simulink model "Furnace"  (R2020a)
settings: Solver=ode15s  StartTime=0  StopTime=12000  FixedStep=0.1  MaxStep=20  RelTol=1e-08  AbsTol=1e-09
undefined symbols (not defined in the file): k, reg
libraries: simulink x9, mpclib x1
(part 2 of 3)

== system Furnace/Plant/Condenser ==
  F_district : Inport
  F_turb : Inport  Port=2
  T_return : Inport  Port=3
  Constant : Constant  Value=k.cp_water
  Constant1 : Constant  Value=k.epsilon_HE
  Constant2 : Constant  Value=k.eff_HE
  District heating heat exchanger : MATLAB Function  TreatAsAtomicUnit=on
  Scope : Scope
  Transport Delay1 : TransportDelay  DelayTime=2
  Transport Delay2 : TransportDelay  DelayTime=2  InitialOutput=k.T_amb  BufferSize=2048
  Transport Delay3 : TransportDelay  DelayTime=2  InitialOutput=k.T_amb
  Transport Delay4 : TransportDelay  DelayTime=2  InitialOutput=k.T_amb
  p_HP : Constant  Value=k.p_HP
  T_district : Outport  VectorParamsAs1DForOutWhenUnconnected=off
  T_w_out : Outport  Port=2  VectorParamsAs1DForOutWhenUnconnected=off
  F_cond : Outport  Port=3  VectorParamsAs1DForOutWhenUnconnected=off
  wires:
  F_district/1 -> District heating heat exchanger/1(F_DH)
  p_HP/1 -> District heating heat exchanger/2(p_HP)
  T_return/1 -> District heating heat exchanger/4(T_return)
  Constant/1 -> District heating heat exchanger/5(cp_water)
  Constant1/1 -> District heating heat exchanger/6(epsilon_HE)
  District heating heat exchanger/1(Q_HE) -> Transport Delay1/1
  District heating heat exchanger/3(T_district) -> Transport Delay3/1
  District heating heat exchanger/2(Tw_ECO) -> Transport Delay2/1
  F_turb/1 -> Transport Delay4/1, District heating heat exchanger/3(F_turb)
  Transport Delay1/1 -> Scope/1
  Transport Delay2/1 -> T_w_out/1
  Transport Delay3/1 -> T_district/1
  Constant2/1 -> District heating heat exchanger/7(eff_HE)
  Transport Delay4/1 -> F_cond/1

== system Furnace/Plant/Flue-gas fan ==
  T_fg : Inport
  Fi_fg : Inport  Port=2
  Fan : MATLAB Function  TreatAsAtomicUnit=on
  Sum of Elements : Sum  Inputs=+
  Out1 : Outport  VectorParamsAs1DForOutWhenUnconnected=off
  Out2 : Outport  Port=2  VectorParamsAs1DForOutWhenUnconnected=off
  tag scope: W_fan=global
  wires:
  T_fg/1 -> Fan/1(T_fg)
  Sum of Elements/1 -> Fan/2(F_fg)
  Fi_fg/1 -> Out2/1, Sum of Elements/1
  Fan/1(T_out) -> Out1/1
  Fan/2(W_el) -> [W_fan]

== system Furnace/Plant/Flue-gas stack ==
  T_fg : Inport
  Fi_fg : Inport  Port=2
  F_fg : Scope
  T_fg_fromECO : Scope
  wires:
  T_fg/1 -> T_fg_fromECO/1
  Fi_fg/1 -> F_fg/1

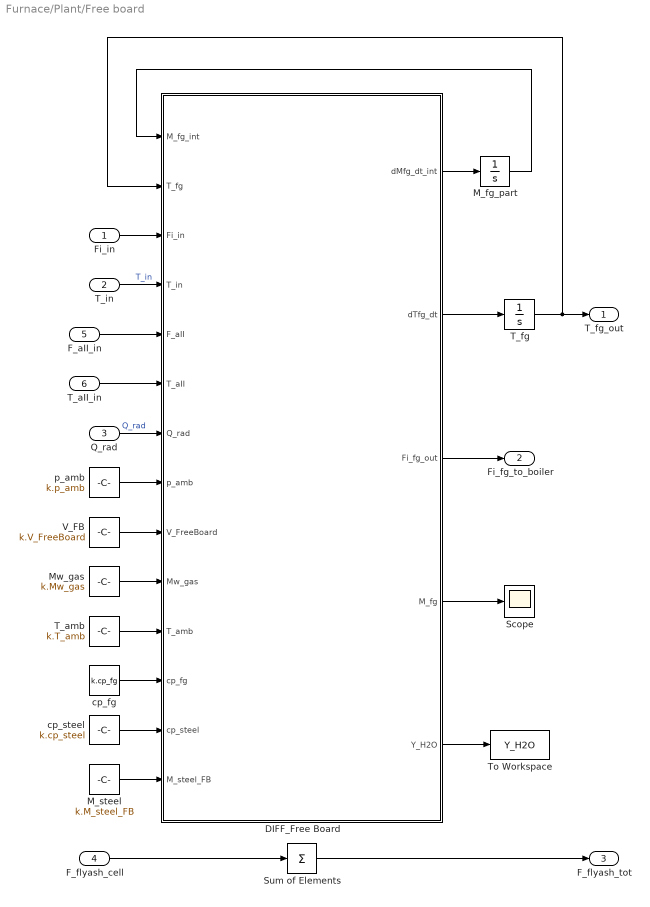
== system Furnace/Plant/Free board ==
  Fi_in : Inport
  T_in : Inport  Port=2
  Q_rad : Inport  Port=3
  F_flyash_cell : Inport  Port=4
  F_aII_in : Inport  Port=5
  T_aII_in : Inport  Port=6
  DIFF_Free Board : MATLAB Function  TreatAsAtomicUnit=on
  M_fg_part : Integrator  InitialCondition=[k.M_fg_IC.*k.w_a(1:k.nc_gas-1)]
  M_steel : Constant  Value=k.M_steel_FB
  Mw_gas : Constant  Value=k.Mw_gas
  Scope : Scope
  Sum of Elements : Sum  Inputs=+
  T_amb : Constant  Value=k.T_amb
  T_fg : Integrator  InitialCondition=k.T_0
  To Workspace : ToWorkspace  VariableName=Y_H2O  SaveFormat=Structure With Time  SampleTime=-1
  V_FB : Constant  Value=k.V_FreeBoard
  cp_fg : Constant  Value=k.cp_fg
  cp_steel : Constant  Value=k.cp_steel
  p_amb : Constant  Value=k.p_amb
  T_fg_out : Outport  VectorParamsAs1DForOutWhenUnconnected=off
  Fi_fg_to_boiler : Outport  Port=2  VectorParamsAs1DForOutWhenUnconnected=off
  F_flyash_tot : Outport  Port=3  VectorParamsAs1DForOutWhenUnconnected=off
  wires:
  T_in/1 -> DIFF_Free Board/4(T_in)  "T_in"
  p_amb/1 -> DIFF_Free Board/8(p_amb)
  DIFF_Free Board/1(dMfg_dt_int) -> M_fg_part/1
  DIFF_Free Board/2(dTfg_dt) -> T_fg/1
  M_fg_part/1 -> DIFF_Free Board/1(M_fg_int)
  DIFF_Free Board/4(M_fg) -> Scope/1
  Q_rad/1 -> DIFF_Free Board/7(Q_rad)  "Q_rad"
  Fi_in/1 -> DIFF_Free Board/3(Fi_in)
  DIFF_Free Board/5(Y_H2O) -> To Workspace/1
  T_fg/1 -> DIFF_Free Board/2(T_fg), T_fg_out/1
  DIFF_Free Board/3(Fi_fg_out) -> Fi_fg_to_boiler/1
  V_FB/1 -> DIFF_Free Board/9(V_FreeBoard)
  Mw_gas/1 -> DIFF_Free Board/10(Mw_gas)
  T_amb/1 -> DIFF_Free Board/11(T_amb)
  cp_fg/1 -> DIFF_Free Board/12(cp_fg)
  cp_steel/1 -> DIFF_Free Board/13(cp_steel)
  M_steel/1 -> DIFF_Free Board/14(M_steel_FB)
  F_flyash_cell/1 -> Sum of Elements/1
  Sum of Elements/1 -> F_flyash_tot/1
  F_aII_in/1 -> DIFF_Free Board/5(F_aII)
  T_aII_in/1 -> DIFF_Free Board/6(T_aII)

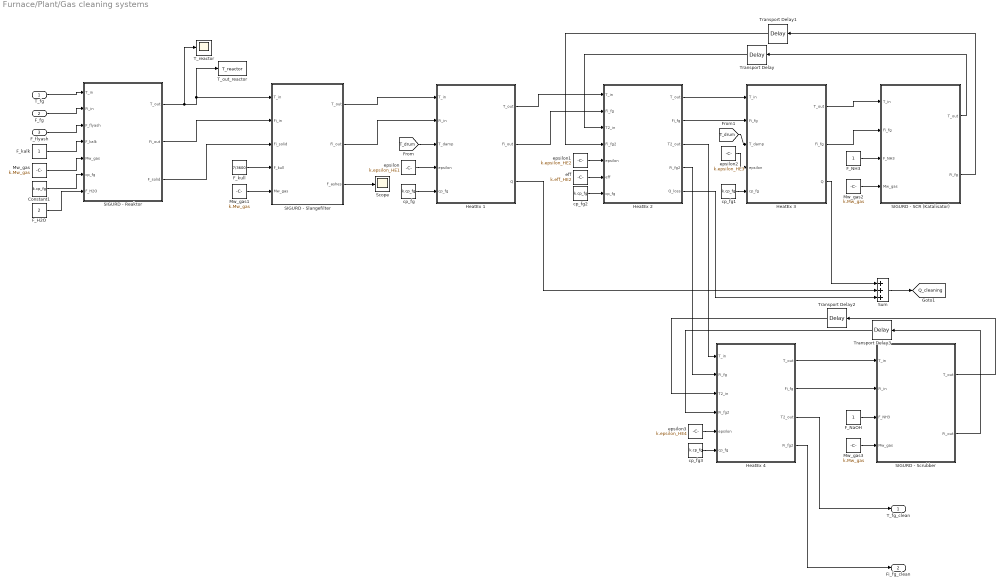
== system Furnace/Plant/Gas cleaning systems ==
  T_fg : Inport
  F_fg : Inport  Port=2
  F_flyash : Inport  Port=3
  Constant1 : Constant  Value=k.cp_fg
  F_H2O : Constant  Value=2
  F_NH3 : Constant
  F_NaOH : Constant
  F_kalk : Constant
  F_kull : Constant  Value=7/3600
  HeatEx 1 : MATLAB Function  TreatAsAtomicUnit=on
  HeatEx 2 : MATLAB Function  TreatAsAtomicUnit=on
  HeatEx 3 : MATLAB Function  TreatAsAtomicUnit=on
  HeatEx 4 : MATLAB Function  TreatAsAtomicUnit=on
  Mw_gas{,1..3} (4 alike) : Constant  Value=k.Mw_gas
  SIGURD - Reaktor : MATLAB Function  TreatAsAtomicUnit=on
  SIGURD - SCR (Katalisator) : MATLAB Function  TreatAsAtomicUnit=on
  SIGURD - Scrubber : MATLAB Function  TreatAsAtomicUnit=on
  SIGURD - Slangefilter : MATLAB Function  TreatAsAtomicUnit=on
  Scope : Scope
  Sum : Sum  Inputs=+++
  T_out_reactor : ToWorkspace  VariableName=T_reactor  SaveFormat=Timeseries  SampleTime=-1
  T_reactor : Scope
  Transport Delay : TransportDelay  DelayTime=2  InitialOutput=k.T_amb
  Transport Delay1 : TransportDelay  DelayTime=2  InitialOutput=ones(k.nc_gas,1)
  Transport Delay2 : TransportDelay  DelayTime=2  InitialOutput=k.T_amb
  Transport Delay3 : TransportDelay  DelayTime=2  InitialOutput=ones(k.nc_gas,1)
  cp_fg{,1..3} (4 alike) : Constant  Value=k.cp_fg
  eff : Constant  Value=k.eff_HE2
  epsilon : Constant  Value=k.epsilon_HE1
  epsilon1 : Constant  Value=k.epsilon_HE2
  epsilon2 : Constant  Value=k.epsilon_HE3
  epsilon3 : Constant  Value=k.epsilon_HE4
  T_fg_clean : Outport  VectorParamsAs1DForOutWhenUnconnected=off
  Fi_fg_clean : Outport  Port=2  VectorParamsAs1DForOutWhenUnconnected=off
  tag scope: Q_cleaning=global
  wires:
  T_fg/1 -> SIGURD - Reaktor/1(T_in)
  F_fg/1 -> SIGURD - Reaktor/2(Fi_in)
  SIGURD - Reaktor/1(T_out) -> T_reactor/1, T_out_reactor/1, SIGURD - Slangefilter/1(T_in)
  SIGURD - Reaktor/2(Fi_out) -> SIGURD - Slangefilter/2(Fi_in)
  F_kalk/1 -> SIGURD - Reaktor/4(F_kalk)
  Mw_gas/1 -> SIGURD - Reaktor/5(Mw_gas)
  F_kull/1 -> SIGURD - Slangefilter/4(F_kull)
  Mw_gas1/1 -> SIGURD - Slangefilter/5(Mw_gas)
  SIGURD - Slangefilter/1(T_out) -> HeatEx 1/1(T_in)
  SIGURD - Slangefilter/2(Fi_out) -> HeatEx 1/2(Fi_in)
  [T_drum] -> HeatEx 1/3(T_damp)
  epsilon/1 -> HeatEx 1/4(epsilon)
  HeatEx 1/1(T_out) -> HeatEx 2/1(T_in)
  HeatEx 1/2(Fi_out) -> HeatEx 2/2("Fi_fg ")
  HeatEx 2/1(T_out) -> HeatEx 3/1(T_in)
  HeatEx 2/2(Fi_fg) -> HeatEx 3/2("Fi_fg ")
  [T_drum] -> HeatEx 3/3(T_damp)
  epsilon1/1 -> HeatEx 2/5(epsilon)
  epsilon2/1 -> HeatEx 3/4(epsilon)
  HeatEx 1/3(Q) -> Sum/2
  HeatEx 3/3(Q) -> Sum/1
  HeatEx 3/1(T_out) -> SIGURD - SCR (Katalisator)/1(T_in)
  HeatEx 3/2(Fi_fg) -> SIGURD - SCR (Katalisator)/2("Fi_fg ")
  F_NH3/1 -> SIGURD - SCR (Katalisator)/3(F_NH3)
  Mw_gas2/1 -> SIGURD - SCR (Katalisator)/4(Mw_gas)
  SIGURD - SCR (Katalisator)/1(T_out) -> Transport Delay/1
  SIGURD - SCR (Katalisator)/2(Fi_fg) -> Transport Delay1/1
  HeatEx 2/3(T2_out) -> HeatEx 4/1(T_in)
  HeatEx 2/4(Fi_fg2) -> HeatEx 4/2("Fi_fg ")
  epsilon3/1 -> HeatEx 4/5(epsilon)
  HeatEx 4/1(T_out) -> SIGURD - Scrubber/1(T_in)
  HeatEx 4/2(Fi_fg) -> SIGURD - Scrubber/2(Fi_in)
  SIGURD - Scrubber/1(T_out) -> Transport Delay2/1
  SIGURD - Scrubber/2(Fi_out) -> Transport Delay3/1
  F_NaOH/1 -> SIGURD - Scrubber/3(F_NH3)
  Mw_gas3/1 -> SIGURD - Scrubber/4(Mw_gas)
  HeatEx 4/3(T2_out) -> T_fg_clean/1
  HeatEx 4/4(Fi_fg2) -> Fi_fg_clean/1
  SIGURD - Slangefilter/3(F_ashes) -> Scope/1
  cp_fg/1 -> HeatEx 1/5(cp_fg)
  cp_fg1/1 -> HeatEx 3/5(cp_fg)
  cp_fg2/1 -> HeatEx 2/7(cp_fg)
  Constant1/1 -> SIGURD - Reaktor/6(cp_fg)
  SIGURD - Reaktor/3(F_solid) -> SIGURD - Slangefilter/3(Fi_solid)
  F_flyash/1 -> SIGURD - Reaktor/3(F_flyash)
  Transport Delay/1 -> HeatEx 2/3(T2_in)
  Transport Delay1/1 -> HeatEx 2/4("Fi_fg2 ")
  Transport Delay2/1 -> HeatEx 4/3(T2_in)
  Transport Delay3/1 -> HeatEx 4/4("Fi_fg2 ")
  cp_fg3/1 -> HeatEx 4/6(cp_fg)
  eff/1 -> HeatEx 2/6(eff)
  Sum/1 -> [Q_cleaning]
  HeatEx 2/5(Q_loss) -> Sum/3
  F_H2O/1 -> SIGURD - Reaktor/7(F_H2O)

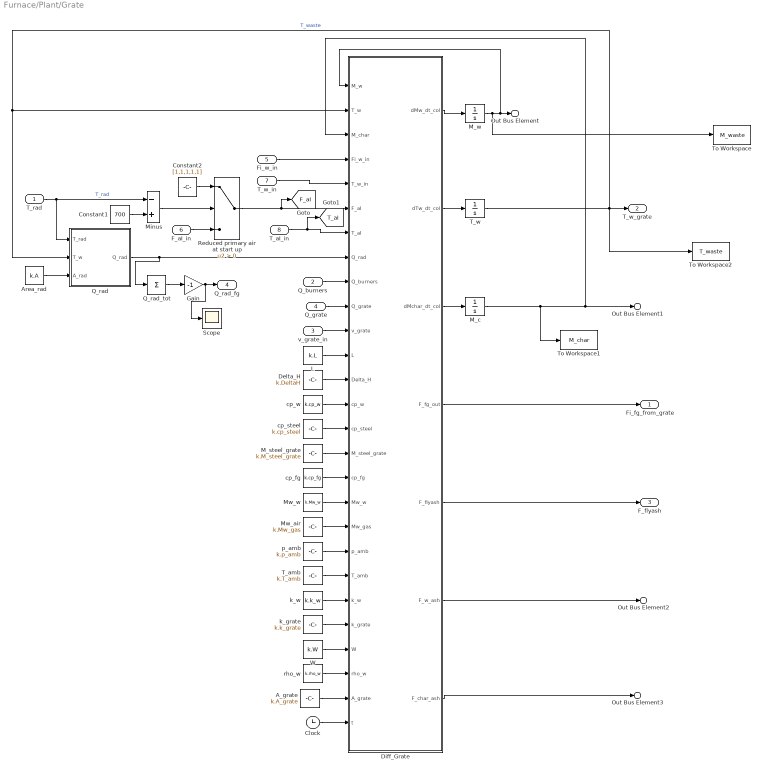
== system Furnace/Plant/Grate ==
  T_rad : Inport
  Q_burners : Inport  Port=2
  v_grate_in : Inport  Port=3
  Q_grate : Inport  Port=4
  Fi_w_in : Inport  Port=5
  F_aI_in : Inport  Port=6
  T_w_in : Inport  Port=7
  T_aI_in : Inport  Port=8
  A_grate : Constant  Value=k.A_grate
  Area_rad : Constant  Value=k.A
  Clock : Clock
  Constant1 : Constant  Value=700
  Constant2 : Constant  Value=[1,1,1,1,1]
  Delta_H : Constant  Value=k.DeltaH
  Diff_Grate : MATLAB Function  TreatAsAtomicUnit=on
  Gain : Gain  Gain=-1
  L : Constant  Value=k.L
  M_c : Integrator  InitialCondition=zeros(k.n_cell,1)
  M_steel_grate : Constant  Value=k.M_steel_grate
  M_w : Integrator  InitialCondition=zeros(k.n_cell.*(k.nc_w+2),1)
  Minus : Sum  Inputs=-+
  Mw_air : Constant  Value=k.Mw_gas
  Mw_w : Constant  Value=k.Mw_w
  Q_rad : Subsystem
  Q_rad_tot : Sum  Inputs=+
  Reduced primary air at start up : Switch  Criteria=u2 > Threshold
  Scope : Scope
  T_amb : Constant  Value=k.T_amb
  T_w : Integrator  InitialCondition=k.T_amb.*ones(k.n_cell,1)
  To Workspace : ToWorkspace  VariableName=M_waste  SaveFormat=Structure With Time  SampleTime=-1
  To Workspace1 : ToWorkspace  VariableName=M_char  SaveFormat=Structure With Time  SampleTime=-1
  To Workspace2 : ToWorkspace  VariableName=T_waste  SaveFormat=Structure With Time  SampleTime=-1
  W : Constant  Value=k.W
  cp_fg : Constant  Value=k.cp_fg
  cp_steel : Constant  Value=k.cp_steel
  cp_w : Constant  Value=k.cp_w
  k_grate : Constant  Value=k.k_grate
  k_w : Constant  Value=k.k_w
  p_amb : Constant  Value=k.p_amb
  rho_w : Constant  Value=k.rho_w
  Fi_fg_from_grate : Outport  VectorParamsAs1DForOutWhenUnconnected=off
  T_w_grate : Outport  Port=2  VectorParamsAs1DForOutWhenUnconnected=off
  F_flyash : Outport  Port=3  VectorParamsAs1DForOutWhenUnconnected=off
  Q_rad_fg : Outport  Port=4  VectorParamsAs1DForOutWhenUnconnected=off
  Out Bus Element : Outport  Port=5  VectorParamsAs1DForOutWhenUnconnected=off  PortName=OutBus  Element=M_w_grate
  Out Bus Element1 : Outport  Port=5  VectorParamsAs1DForOutWhenUnconnected=off  PortName=OutBus  Element=M_char
  Out Bus Element2 : Outport  Port=5  VectorParamsAs1DForOutWhenUnconnected=off  PortName=OutBus  Element=F_w_ash
  Out Bus Element3 : Outport  Port=5  VectorParamsAs1DForOutWhenUnconnected=off  PortName=OutBus  Element=F_char_ash
  tag scope: F_aI=global, T_aI=global
  wires:
  Diff_Grate/2(dTw_dt_col) -> T_w/1
  Area_rad/1 -> Q_rad/3(A_rad)
  M_w/1 -> To Workspace/1, Out Bus Element/1, Diff_Grate/1(M_w)
  T_aI_in/1 -> [T_aI], Diff_Grate/7(T_aI)
  Q_rad/1(Q_rad) -> Q_rad_tot/1, Diff_Grate/8(Q_rad)
  Diff_Grate/1(dMw_dt_col) -> M_w/1
  T_w/1 -> Diff_Grate/2(T_w), Q_rad/2(T_w), T_w_grate/1, To Workspace2/1  "T_waste"
  Diff_Grate/6(F_w_ash) -> Out Bus Element2/1
  Diff_Grate/4(F_fg_out) -> Fi_fg_from_grate/1
  Diff_Grate/3(dMchar_dt_col) -> M_c/1
  M_c/1 -> To Workspace1/1, Out Bus Element1/1, Diff_Grate/3(M_char)
  Diff_Grate/7(F_char_ash) -> Out Bus Element3/1
  Q_rad_tot/1 -> Gain/1
  Gain/1 -> Scope/1, Q_rad_fg/1
  Q_burners/1 -> Diff_Grate/9(Q_burners)
  Clock/1 -> Diff_Grate/27(t)
  Q_grate/1 -> Diff_Grate/10(Q_grate)
  T_rad/1 -> Minus/1, Q_rad/1(T_rad)  "T_rad"
  Constant1/1 -> Minus/2
  Minus/1 -> Reduced primary air at start up/2
  F_aI_in/1 -> Reduced primary air at start up/3
  Reduced primary air at start up/1 -> [F_aI], Diff_Grate/6(F_aI)
  Constant2/1 -> Reduced primary air at start up/1
  L/1 -> Diff_Grate/12(L)
  Delta_H/1 -> Diff_Grate/13(Delta_H)
  cp_w/1 -> Diff_Grate/14(cp_w)
  cp_steel/1 -> Diff_Grate/15(cp_steel)
  M_steel_grate/1 -> Diff_Grate/16(M_steel_grate)
  cp_fg/1 -> Diff_Grate/17(cp_fg)
  Mw_w/1 -> Diff_Grate/18(Mw_w)
  Mw_air/1 -> Diff_Grate/19(Mw_gas)
  p_amb/1 -> Diff_Grate/20(p_amb)
  T_amb/1 -> Diff_Grate/21(T_amb)
  k_w/1 -> Diff_Grate/22(k_w)
  k_grate/1 -> Diff_Grate/23(k_grate)
  W/1 -> Diff_Grate/24(W)
  rho_w/1 -> Diff_Grate/25(rho_w)
  A_grate/1 -> Diff_Grate/26(A_grate)
  Diff_Grate/5(F_flyash) -> F_flyash/1
  v_grate_in/1 -> Diff_Grate/11(v_grate)
  Fi_w_in/1 -> Diff_Grate/4(Fi_w_in)
  T_w_in/1 -> Diff_Grate/5(T_w_in)

== system Furnace/Plant/Hot water to district heating ==
  In1 : Inport
  T_district : Scope
  wires:
  In1/1 -> T_district/1

== system Furnace/Plant/Turbine ==
  T_SH : Inport
  F_SH : Inport  Port=2
  p_drum : Inport  Port=3
  Scope : Scope
  Sum : Sum
  Transport Delay1 : TransportDelay  DelayTime=3
  Transport Delay2 : TransportDelay  DelayTime=3
  Turbine : MATLAB Function  TreatAsAtomicUnit=on
  W_net : Scope
  eta_TURB : Constant  Value=k.eta_TURB
  p_HP : Constant  Value=k.p_HP
  p_LP : Constant  Value=k.p_LP
  F_turb : Outport  VectorParamsAs1DForOutWhenUnconnected=off
  wires:
  T_SH/1 -> Turbine/1(T_SH)
  Turbine/1(W_el) -> Transport Delay1/1
  p_drum/1 -> Turbine/3(p_drum)
  F_SH/1 -> Transport Delay2/1, Turbine/2(F_SH)
  p_LP/1 -> Turbine/5(p_LP)
  Transport Delay1/1 -> Sum/1
  Transport Delay2/1 -> F_turb/1
  p_HP/1 -> Turbine/4(p_HP)
  Turbine/2(Q_turb) -> Scope/1
  eta_TURB/1 -> Turbine/6(eta_TURB)
  [W_fan] -> Sum/2
  Sum/1 -> W_net/1

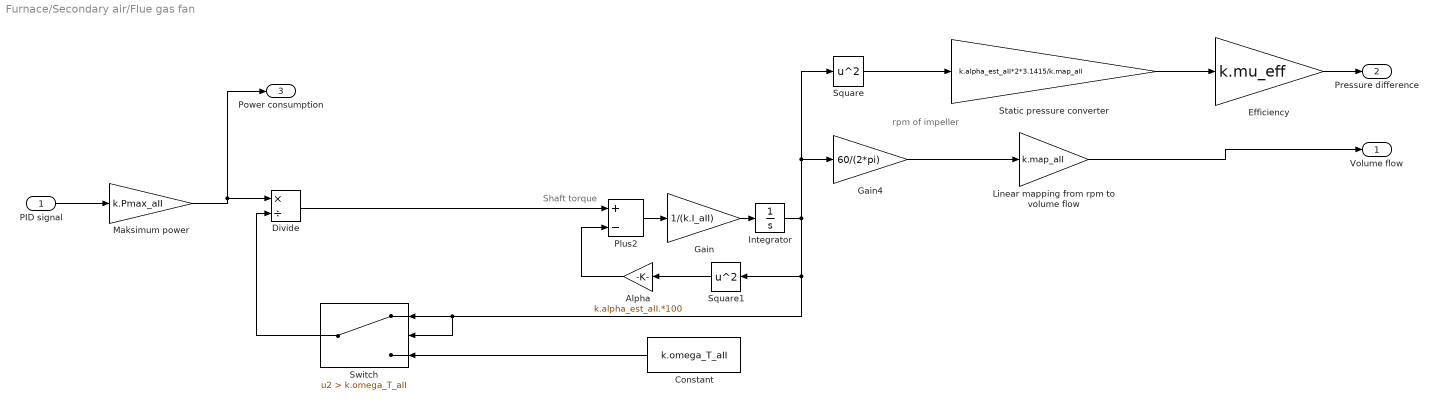
== system Furnace/Secondary air/Flue gas fan ==
  note: rpm of impeller
  note: Shaft torque
  PID signal : Inport
  Alpha : Gain  Gain=k.alpha_est_aII.*100
  Constant : Constant  Value=k.omega_T_aII
  Divide : Product  Inputs=*/
  Efficiency : Gain  Gain=k.mu_eff
  Gain : Gain  Gain=1/(k.I_aII)
  Gain4 : Gain  Gain=60/(2*pi)
  Integrator : Integrator  InitialCondition=reg.F_aII_fan_model_int
  "Linear mapping from rpm to volume flow " : Gain  Gain=k.map_aII
  "Maksimum power " : Gain  Gain=k.Pmax_aII
  Plus2 : Sum  Inputs=+-
  Square : Math  Operator=square  SignedPower=on  SaturateOnIntegerOverflow=on
  Square1 : Math  Operator=square  SignedPower=on  SaturateOnIntegerOverflow=on
  Static pressure converter : Gain  Gain=k.alpha_est_aII*2*3.1415/k.map_aII
  Switch : Switch  Criteria=u2 > Threshold  Threshold=k.omega_T_aII
  Volume flow : Outport  VectorParamsAs1DForOutWhenUnconnected=off
  Pressure difference : Outport  Port=2  VectorParamsAs1DForOutWhenUnconnected=off
  Power consumption : Outport  Port=3  VectorParamsAs1DForOutWhenUnconnected=off
  wires:
  Integrator/1 -> Square/1, Gain4/1, Switch/2, Switch/1, Square1/1
  Divide/1 -> Plus2/1
  Gain4/1 -> "Linear mapping from rpm to volume flow "/1
  Square/1 -> Static pressure converter/1
  Efficiency/1 -> Pressure difference/1
  "Maksimum power "/1 -> Power consumption/1, Divide/1
  Static pressure converter/1 -> Efficiency/1
  Alpha/1 -> Plus2/2
  Square1/1 -> Alpha/1
  Gain/1 -> Integrator/1
  Plus2/1 -> Gain/1
  PID signal/1 -> "Maksimum power "/1
  "Linear mapping from rpm to volume flow "/1 -> Volume flow/1
  Switch/1 -> Divide/2
  Constant/1 -> Switch/3

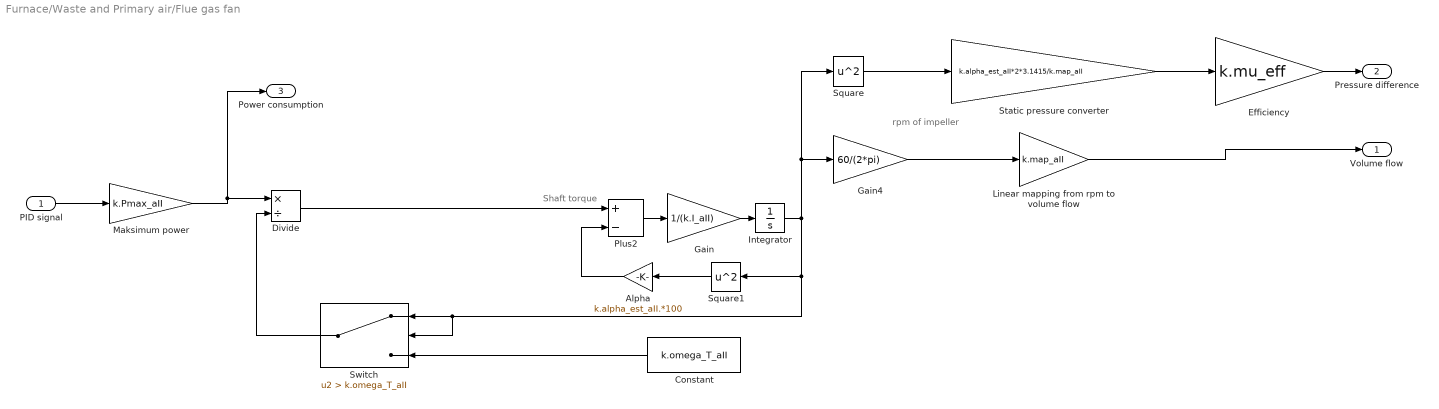
== system Furnace/Waste and Primary air/Flue gas fan ==
  note: rpm of impeller
  note: Shaft torque
  PID signal : Inport
  Alpha : Gain  Gain=k.alpha_est_aII.*100
  Constant : Constant  Value=k.omega_T_aII
  Divide : Product  Inputs=*/
  Efficiency : Gain  Gain=k.mu_eff
  Gain : Gain  Gain=1/(k.I_aII)
  Gain4 : Gain  Gain=60/(2*pi)
  Integrator : Integrator  InitialCondition=reg.F_aI_fan_model_int
  "Linear mapping from rpm to volume flow " : Gain  Gain=k.map_aII
  "Maksimum power " : Gain  Gain=k.Pmax_aII
  Plus2 : Sum  Inputs=+-
  Square : Math  Operator=square  SignedPower=on  SaturateOnIntegerOverflow=on
  Square1 : Math  Operator=square  SignedPower=on  SaturateOnIntegerOverflow=on
  Static pressure converter : Gain  Gain=k.alpha_est_aII*2*3.1415/k.map_aII
  Switch : Switch  Criteria=u2 > Threshold  Threshold=k.omega_T_aII
  Volume flow : Outport  VectorParamsAs1DForOutWhenUnconnected=off
  Pressure difference : Outport  Port=2  VectorParamsAs1DForOutWhenUnconnected=off
  Power consumption : Outport  Port=3  VectorParamsAs1DForOutWhenUnconnected=off
  wires:
  Integrator/1 -> Square/1, Gain4/1, Switch/2, Switch/1, Square1/1
  Divide/1 -> Plus2/1
  Gain4/1 -> "Linear mapping from rpm to volume flow "/1
  Square/1 -> Static pressure converter/1
  Efficiency/1 -> Pressure difference/1
  "Maksimum power "/1 -> Power consumption/1, Divide/1
  Static pressure converter/1 -> Efficiency/1
  Alpha/1 -> Plus2/2
  Square1/1 -> Alpha/1
  Gain/1 -> Integrator/1
  Plus2/1 -> Gain/1
  PID signal/1 -> "Maksimum power "/1
  "Linear mapping from rpm to volume flow "/1 -> Volume flow/1
  Switch/1 -> Divide/2
  Constant/1 -> Switch/3

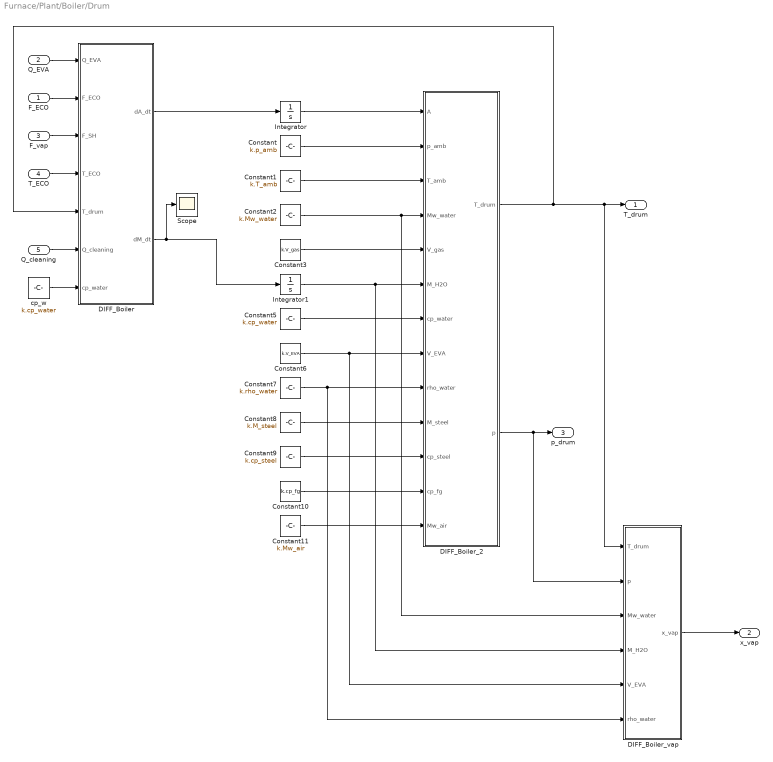
== system Furnace/Plant/Boiler/Drum ==
  F_ECO : Inport
  Q_EVA : Inport  Port=2
  F_vap : Inport  Port=3
  T_ECO : Inport  Port=4
  Q_cleaning : Inport  Port=5
  Constant : Constant  Value=k.p_amb
  Constant1 : Constant  Value=k.T_amb
  Constant10 : Constant  Value=k.cp_fg
  Constant11 : Constant  Value=k.Mw_air
  Constant2 : Constant  Value=k.Mw_water
  Constant3 : Constant  Value=k.V_gas
  Constant5 : Constant  Value=k.cp_water
  Constant6 : Constant  Value=k.V_EVA
  Constant7 : Constant  Value=k.rho_water
  Constant8 : Constant  Value=k.M_steel
  Constant9 : Constant  Value=k.cp_steel
  "DIFF_Boiler " : MATLAB Function  TreatAsAtomicUnit=on
  DIFF_Boiler_2 : MATLAB Function  TreatAsAtomicUnit=on
  DIFF_Boiler_vap : MATLAB Function  TreatAsAtomicUnit=on
  Integrator : Integrator  InitialCondition=k.A_0
  Integrator1 : Integrator  InitialCondition=k.M_H2O
  Scope : Scope
  cp_w : Constant  Value=k.cp_water
  T_drum : Outport  VectorParamsAs1DForOutWhenUnconnected=off
  x_vap : Outport  Port=2  VectorParamsAs1DForOutWhenUnconnected=off
  p_drum : Outport  Port=3  PortDimensions=1  VectorParamsAs1DForOutWhenUnconnected=off
  wires:
  F_vap/1 -> "DIFF_Boiler "/3(F_SH)
  Q_EVA/1 -> "DIFF_Boiler "/1(Q_EVA)
  F_ECO/1 -> "DIFF_Boiler "/2(F_ECO)
  "DIFF_Boiler "/1(dA_dt) -> Integrator/1
  Integrator/1 -> DIFF_Boiler_2/1(A)
  DIFF_Boiler_vap/1(x_vap) -> x_vap/1
  DIFF_Boiler_2/2(p) -> DIFF_Boiler_vap/2(p), p_drum/1
  Constant/1 -> DIFF_Boiler_2/2(p_amb)
  Constant1/1 -> DIFF_Boiler_2/3(T_amb)
  Constant2/1 -> DIFF_Boiler_2/4(Mw_water), DIFF_Boiler_vap/3(Mw_water)
  Constant3/1 -> DIFF_Boiler_2/5(V_gas)
  Integrator1/1 -> DIFF_Boiler_vap/4(M_H2O), DIFF_Boiler_2/6(M_H2O)
  Constant5/1 -> DIFF_Boiler_2/7(cp_water)
  Constant6/1 -> DIFF_Boiler_2/8(V_EVA), DIFF_Boiler_vap/5(V_EVA)
  Constant7/1 -> DIFF_Boiler_2/9(rho_water), DIFF_Boiler_vap/6(rho_water)
  Constant8/1 -> DIFF_Boiler_2/10(M_steel)
  Constant9/1 -> DIFF_Boiler_2/11(cp_steel)
  Constant10/1 -> DIFF_Boiler_2/12(cp_fg)
  Constant11/1 -> DIFF_Boiler_2/13(Mw_air)
  T_ECO/1 -> "DIFF_Boiler "/4(T_ECO)
  DIFF_Boiler_2/1(T_drum) -> "DIFF_Boiler "/5(T_drum), DIFF_Boiler_vap/1(T_drum), T_drum/1
  Q_cleaning/1 -> "DIFF_Boiler "/6(Q_cleaning)
  cp_w/1 -> "DIFF_Boiler "/7(cp_water)
  "DIFF_Boiler "/2(dM_dt) -> Integrator1/1, Scope/1

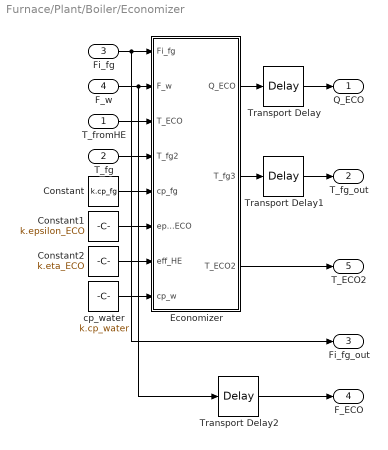
== system Furnace/Plant/Boiler/Economizer ==
  T_fromHE : Inport
  T_fg : Inport  Port=2
  Fi_fg : Inport  Port=3
  F_w : Inport  Port=4
  Constant : Constant  Value=k.cp_fg
  Constant1 : Constant  Value=k.epsilon_ECO
  Constant2 : Constant  Value=k.eta_ECO
  Economizer : MATLAB Function  TreatAsAtomicUnit=on
  Transport Delay : TransportDelay  DelayTime=2
  Transport Delay1 : TransportDelay  DelayTime=2  InitialOutput=k.T_amb
  Transport Delay2 : TransportDelay  DelayTime=2
  cp_water : Constant  Value=k.cp_water
  Q_ECO : Outport  VectorParamsAs1DForOutWhenUnconnected=off
  T_fg_out : Outport  Port=2  VectorParamsAs1DForOutWhenUnconnected=off
  Fi_fg_out : Outport  Port=3  VectorParamsAs1DForOutWhenUnconnected=off
  F_ECO : Outport  Port=4  VectorParamsAs1DForOutWhenUnconnected=off
  T_ECO2 : Outport  Port=5  VectorParamsAs1DForOutWhenUnconnected=off
  wires:
  Fi_fg/1 -> Fi_fg_out/1, Economizer/1(Fi_fg)
  T_fg/1 -> Economizer/4(T_fg2)
  T_fromHE/1 -> Economizer/3(T_ECO)
  Constant/1 -> Economizer/5(cp_fg)
  Constant1/1 -> Economizer/6(epsilon_ECO)
  Economizer/1(Q_ECO) -> Transport Delay/1
  Economizer/2(T_fg3) -> Transport Delay1/1
  F_w/1 -> Transport Delay2/1, Economizer/2(F_w)
  Transport Delay/1 -> Q_ECO/1
  Transport Delay1/1 -> T_fg_out/1
  Constant2/1 -> Economizer/7(eff_HE)
  cp_water/1 -> Economizer/8(cp_w)
  Economizer/3(T_ECO2) -> T_ECO2/1
  Transport Delay2/1 -> F_ECO/1

== system Furnace/Plant/Boiler/Evaporator ==
  T_drum : Inport
  T_fg : Inport  Port=2
  Fi_fg : Inport  Port=3
  Constant : Constant  Value=k.cp_fg
  Constant1 : Constant  Value=k.epsilon_EVA
  Constant2 : Constant  Value=k.eff_HE
  Evaporator : MATLAB Function  TreatAsAtomicUnit=on
  Transport Delay : TransportDelay  DelayTime=5  InitialOutput=k.T_amb
  Q_EVA : Outport  VectorParamsAs1DForOutWhenUnconnected=off
  T_fg_out : Outport  Port=2  VectorParamsAs1DForOutWhenUnconnected=off
  Fi_fg_out : Outport  Port=3  VectorParamsAs1DForOutWhenUnconnected=off
  wires:
  T_drum/1 -> Evaporator/2(T_drum)
  Constant/1 -> Evaporator/4(cp_fg)
  Constant1/1 -> Evaporator/5(epsilon_EVA)
  Evaporator/1(Q_EVA) -> Q_EVA/1
  Evaporator/2(T_fg2) -> Transport Delay/1
  T_fg/1 -> Evaporator/3(T_fg1)
  Fi_fg/1 -> Fi_fg_out/1, Evaporator/1(Fi_fg)
  Transport Delay/1 -> T_fg_out/1
  Constant2/1 -> Evaporator/6(eff_HE)

== system Furnace/Plant/Boiler/Super heater ==
  F_steam : Inport
  T_drum : Inport  Port=2
  T_fg : Inport  Port=3
  Fi_fg : Inport  Port=4
  Constant : Constant  Value=k.cp_fg
  Constant1 : Constant  Value=k.epsilon_SH
  Constant2 : Constant  Value=k.eff_HE
  Super heater : MATLAB Function  TreatAsAtomicUnit=on
  Transport Delay : TransportDelay  DelayTime=2  InitialOutput=k.T_amb
  Transport Delay1 : TransportDelay  DelayTime=2  InitialOutput=k.T_amb
  Transport Delay2 : TransportDelay  DelayTime=2
  Q_SH : Outport  VectorParamsAs1DForOutWhenUnconnected=off
  T_steam : Outport  Port=2  VectorParamsAs1DForOutWhenUnconnected=off
  T_fg_out : Outport  Port=3  VectorParamsAs1DForOutWhenUnconnected=off
  Fi_fg_out : Outport  Port=4  VectorParamsAs1DForOutWhenUnconnected=off
  F_SH : Outport  Port=5  VectorParamsAs1DForOutWhenUnconnected=off
  wires:
  F_steam/1 -> F_SH/1, Super heater/1(F_steam)
  T_drum/1 -> Super heater/3(T_drum)
  T_fg/1 -> Super heater/4(T_fg1)
  Constant/1 -> Super heater/5(cp_fg)
  Constant1/1 -> Super heater/6(epsilon_SH)
  Fi_fg/1 -> Fi_fg_out/1, Super heater/2(Fi_fg)
  Super heater/3(T_fg2) -> Transport Delay/1
  Super heater/2(T_steam) -> Transport Delay1/1
  Super heater/1(Q_SH) -> Transport Delay2/1
  Transport Delay/1 -> T_fg_out/1
  Transport Delay1/1 -> T_steam/1
  Transport Delay2/1 -> Q_SH/1
  Constant2/1 -> Super heater/7(eff_HE)

== system Furnace/Plant/Grate/Q_rad ==
  T_rad : Inport
  T_w : Inport  Port=2
  A_rad : Inport  Port=3
  1/n_cell : Gain  Gain=1./k.n_cell
  "Power " : Constant  Value=4
  Product : Product
  T_rad^4 : Math  Operator=pow  SignedPower=on  OutputSignalType=real  SaturateOnIntegerOverflow=on
  T_w^4 : Math  Operator=pow  SignedPower=on  OutputSignalType=real  SaturateOnIntegerOverflow=on
  "alpha_gt " : Gain  Gain=k.alpha_gt
  epsilon : Gain  Gain=k.epsilon_gt
  sigma : Gain  Gain=k.sigma
  sum : Sum  Inputs=+-
  Q_rad : Outport  VectorParamsAs1DForOutWhenUnconnected=off
  wires:
  A_rad/1 -> 1/n_cell/1
  "Power "/1 -> T_w^4/2, T_rad^4/2
  sigma/1 -> Product/1
  epsilon/1 -> sum/1
  sum/1 -> sigma/1
  T_w^4/1 -> "alpha_gt "/1
  T_rad/1 -> T_rad^4/1
  T_w/1 -> T_w^4/1
  "alpha_gt "/1 -> sum/2
  Product/1 -> Q_rad/1
  T_rad^4/1 -> epsilon/1
  1/n_cell/1 -> Product/2

== matlab function Furnace/Plant/Boiler/Super heater/Super heater ==
  data: Q_SH output; F_steam input; T_steam output size=1; Fi_fg input; T_drum input; T_fg1 input; cp_fg input; epsilon_SH input; T_fg2 output size=1; eff_HE input
function [Q_SH,T_steam,T_fg2] = CALC_Q_SH(F_steam,Fi_fg,T_drum,T_fg1,cp_fg,epsilon_SH,eff_HE)

% This function calculates the heat exchanged in the super heater

F_fg    = sum(Fi_fg); 

if F_steam == 0 
    T_steam = T_drum;
    T_fg2   = T_fg1;
    Q_SH    = 0;
else
    [~,T_sat,~,~,~,c_p]=SatWater;
    cp_steam= interp1(T_sat,c_p,T_drum,'linear','extrap');
    C_min   = min(cp_fg.*F_fg,cp_steam.*F_steam);
    Q_SH    = epsilon_SH.*C_min.*(T_fg1-T_drum);
    T_fg2   = T_fg1 - Q_SH./(cp_fg.*F_fg);
    T_steam =  T_drum + Q_SH./(cp_steam.*F_steam);
end
Q_SH        = Q_SH.*eff_HE;

== matlab function Furnace/Plant/Boiler/Economizer/Economizer ==
  data: Fi_fg input; F_w input; Q_ECO output; T_ECO input; T_fg2 input; cp_fg input; epsilon_ECO input; T_fg3 output; eff_HE input; cp_w input; T_ECO2 output
function [Q_ECO,T_fg3,T_ECO2] = CALC_Q_ECO(Fi_fg,F_w,T_ECO,T_fg2,cp_fg,epsilon_ECO,eff_HE, cp_w)

% This function calculates the heat exchanged in the economizer

F_fg    = sum(Fi_fg);
C_min   = cp_fg.*F_fg;
if F_w == 0 
    Q_ECO   = 0;
    T_fg3   = T_fg2;
    T_ECO2  = T_ECO;
else
    Q_ECO   = epsilon_ECO.*C_min.*(T_fg2-T_ECO);
    T_fg3   = T_fg2 - Q_ECO./(cp_fg.*F_fg);
    T_ECO2  = T_ECO + Q_ECO.*eff_HE./(cp_w.*F_w);
end
Q_ECO       = Q_ECO.*eff_HE;

== matlab function Furnace/Plant/Condenser/District heating heat exchanger ==
  data: F_DH input; Q_HE output; p_HP input; F_turb input; T_return input; cp_water input; epsilon_HE input; Tw_ECO output; T_district output; eff_HE input
function [Q_HE,Tw_ECO,T_district] = CALC_Q_HE(F_DH,p_HP,F_turb,T_return,cp_water,epsilon_HE,eff_HE)

% This function calculates the heat exchanged between the steam from the
% drum and the water from the district heating net
C_min   = cp_water.*F_DH;
[p_sat,T_sat,~,~,~,~] = SatWater;
T_HP    = interp1(p_sat,T_sat,p_HP,'linear','extrap');
if F_turb == 0
    Q_HE    = 0;
else 
    
    Q_HE    = epsilon_HE.*C_min.*(T_HP-T_return);
end
Tw_ECO      = T_HP;
T_district  = T_return + Q_HE./C_min;
Q_HE        = Q_HE./eff_HE;

== matlab function Furnace/Plant/Boiler/Drum/DIFF_Boiler  ==
  data: Q_EVA input; dA_dt output size=1; F_ECO input; F_SH input; T_ECO input; T_drum input; Q_cleaning input; cp_water input; dM_dt output
function [dA_dt,dM_dt]  = DIFF_Boiler(Q_EVA ,F_ECO, F_SH,T_ECO, T_drum, Q_cleaning,cp_water)

% Energy in the drum [J]
%% ENERGY BALANCE EQUATION
[~,T_sat,~,h_w,h_vap,~] = SatWater;
if T_drum < 373.15
    dA_dt   = Q_EVA - Q_cleaning;
    dM_dt   = 0;
else
    % Enthalpy of water vapor at T_drum [J/kg]
    h_steam = interp1(T_sat,h_vap,T_drum,'linear','extrap');
    % Enthalpy of water at T_drum [J/kg]
    h_water = interp1(T_sat,h_w,T_drum,'linear','extrap');
    h_ECO   = h_water - cp_water.*(T_drum-T_ECO);
    % Energy balance
    dA_dt   = Q_EVA - F_SH.*h_steam  + F_ECO.*h_ECO - Q_cleaning;
    dM_dt   = - F_SH + F_ECO;
end

== matlab function Furnace/Plant/Boiler/Drum/DIFF_Boiler_2 ==
  data: A input; T_drum output; p_amb input; T_amb input; Mw_water input; V_gas input; M_H2O input; cp_water input; V_EVA input; rho_water input; M_steel input; cp_steel input; cp_fg input; Mw_air input; p output
function [T_drum,p] = Boiler(A,p_amb,T_amb,Mw_water,V_gas,M_H2O,cp_water,V_EVA,rho_water,M_steel,cp_steel,cp_fg,Mw_air)

% This function calculates the pressure and temperature in the boiler drum
% from the total energy in the drum. The start up description should be
% changed when we know how boiler start up actually works.

%%%%%%%%%%%%%%%%%%%%%%%%%%%%%%%%%%%%%%%%%%%%%%%%%%%%%%%%%%%%%%%%%%%%%%%%%%%
% Symbol        Units       Explanation
% INPUTS:
% A             [J]         Energy stored in the boiler drum
% p_amb         [Pa]        Ambient pressure
% T_amb         [K]         Ambient temperature
% Mw_water      [kg/kmol]   Molar weight of water
% V_gas         [m3]        Volume of drum boiler initilly occupied by air
% M_H2O         [kg]        Mass of water in the boiler
% cp_water      [J/kg K]    Specific heat capacity of water
% V_EVA         [m3]        Total volume of boiler
% rho_water     [kg/m3]     Density of water
% M_steel       [kg]        Total mass of steel in the boiler
% cp_steel      [J/kg K]    Specific heat capacity of steel
% cp_fg         [J/kg K]    Specific heat capicity of fuel gasses
% Mw_air        [kg/kmol]   Molar weight of air/fuel gasses
%%%%%%%%%%%%%%%%%%%%%%%%%%%%%%%%%%%%%%%%%%%%%%%%%%%%%%%%%%%%%%%%%%%%%%%%%%%

% Energy in the drum [J]
A_en        = A;
R           = 8.314462175*1E3;
%% ENERGY BALANCE EQUATION
[p_sat,T_sat,rho_vap,h_w,h_vap,~] = SatWater;
T_drum      = fzero(@find_T,273);
if T_drum < 373.15
    p  	= p_amb;
else
    p   = interp1(T_sat,p_sat,T_drum,'linear','extrap');
end

%%%%%%%%%%%%%%%%%%%%%%%%%%%%%%%%%%%%%%%%%%%%%%%%%%%%%%%%%%%%%%%%%%%%%%%%%%%
% This subfunction finds the temperature of the drum that satisfies the
% energy balance. We assume that the cold boiler is initially filled with
% water (M_H2O) and air (which occupies the volume V_gas). The boiler has a
% valve, which is open as long as T_drum<373.15K, so that the air can be
% discharged in the atmosphere as the boiler warms up and the water
% eveporates. In this way, the pressure is mantained at p=p_amb. When
% T_drum reaches 373.15K, the valve closes and pressure builds up as the
% water starts evaporating, so that saturated water and steam are always
% present in the vessel, at the relative saturated temperature and pressure

    function Res    = find_T(X)
        T_drum      = X;
        if T_drum < 373.15
            % When T_drum<375.15K, the valve is open and p=p_amb [Pa]
            p       = p_amb;
            % The air is assumed to be saturated with water [kmol_vap/kmol]
            y_sat   = CALC_xsat(T_drum);
            % Partial pressure of water vapor [Pa]
            p_vap   = y_sat*p;
            % Specific entalphy of water at 373.15K [J/kg]
            h_w_sat = interp1(T_sat,h_w,373.15,'linear','extrap');
            % Enthalpy of water at T_drum [J/kg]
            h_water = h_w_sat - cp_water.*(373.15-T_drum);
            % Enthalpy of water vapor at T_drum [J/kg]
            h_steam = interp1(T_sat,h_vap,T_drum,'linear','extrap');
            % Vapor fraction
            x_vap   = fzero(@find_x_vap,0);
            % Moles of air in the drum [kmol]
            N_air   = (p-p_vap).*V_gas./(R.*T_drum);
            % Mass of air in the drum [kg]
            M_air   = N_air.*Mw_air;
        else
            % Enthalpy of water vapor at T_drum [J/kg]
            h_steam = interp1(T_sat,h_vap,T_drum,'linear','extrap');
            % Enthalpy of water at T_drum [J/kg]
            h_water = interp1(T_sat,h_w,T_drum,'linear','extrap');
            % Pressure of boiling water at T_drum [Pa]
            p       = interp1(T_sat,p_sat,T_drum,'linear','extrap');
            % Find the vapor fraction
            x_vap   = fzero(@find_x_vap,0);
            % No air is left in the boiler after start up
            M_air   = 0;
        end

        Res         = A_en- (M_H2O.*x_vap.*h_steam + M_H2O.*(1-x_vap).*h_water -p.*V_EVA + M_steel.*cp_steel.*(T_drum-T_amb) + M_air.*cp_fg.*(T_drum-T_amb));
    end
%%%%%%%%%%%%%%%%%%%%%%%%%%%%%%%%%%%%%%%%%%%%%%%%%%%%%%%%%%%%%%%%%%%%%%%%%%%
    function Res = find_x_vap(Y)
        x_vap   = Y;
        M_vap   = x_vap.*M_H2O;
        if T_drum < 373.15
            y_sat   = CALC_xsat(T_drum);
            p_vap   = y_sat*p_amb;
            V_vap   = V_EVA - (M_H2O-M_vap)./rho_water;
            Res     = (M_vap-p_vap.*V_vap./(R.*T_drum).*Mw_water);
        else
            % Density of saturated vapor at T_drum [kg/m3]
            rho_steam   = interp1(T_sat,rho_vap,T_drum,'linear','extrap');
            % Compressibility factor of vapor [-]
            Z_steam     = p.*Mw_water./(rho_steam.*R.*T_drum);
            % Moles of water vapor [kmol]
            N_steam     = M_H2O.*x_vap./Mw_water;
            % Pressure calculated from the vapor fraction [Pa]
            V_steam     = V_EVA-(1-x_vap).*M_H2O./rho_water;
            p2          = Z_steam.*N_steam.*R.*T_drum./V_steam;
            % p2 should be the same as p
            Res     = (p-p2);
        end
    end
end

== matlab function Furnace/Plant/Boiler/Drum/DIFF_Boiler_vap ==
  data: T_drum input; x_vap output; p input; Mw_water input; M_H2O input; V_EVA input; rho_water input
function x_vap  = Boiler_vap(T_drum,p,Mw_water,M_H2O,V_EVA,rho_water)

R           = 8.314462175*1E3;
%% ENERGY BALANCE EQUATION
x_vap = fzero(@find_x_vap,0);

%%%%%%%%%%%%%%%%%%%%%%%%%%%%%%%%%%%%%%%%%%%%%%%%%%%%%%%%%%%%%%%%%%%%%%%%%%%
    function Res    = find_x_vap(Y)
        x_vap       = Y;
        M_vap       = x_vap.*M_H2O;
        if T_drum < 373.15
            y_sat   = CALC_xsat(T_drum);
            p_vap   = y_sat*p;
            V_vap   = V_EVA - (M_H2O-M_vap)./rho_water;
            Res    = (M_vap-p_vap.*V_vap./(R.*T_drum).*Mw_water);
        else
            [~,T_sat,rho_vap,~,~,~] = SatWater;
            % Density of saturated vapor at T_drum [kg/m3]
            rho_steam   = interp1(T_sat,rho_vap,T_drum,'linear','extrap');
            % Compressibility factor of vapor [-]
            Z_steam     = p.*Mw_water./(rho_steam.*R.*T_drum);
            % Moles of water vapor [kmol]
            N_steam     = M_H2O.*x_vap./Mw_water;
            % Pressure calculated from the vapor fraction [Pa]
            V_steam     = V_EVA-(1-x_vap).*M_H2O./rho_water;
            p2          = Z_steam.*N_steam.*R.*T_drum./V_steam;
            % p2 should be the same as p
            Res         = (p-p2);
        end
    end
end
% function x  = Boiler_vap(T_drum,p,p_amb,Mw_water,V_gas,M_H2O,V_EVA,rho_water)
% 
% R           = 8.314462175*1E3;
% %% ENERGY BALANCE EQUATION
% [p_sat,T_sat,rho_vap,~,~,~] = SatWater;
% x   = fzero(@find_x_vap,0);
% 
% 
% function Res = find_x_vap(Y)
% x_vap   = Y;
% if T_drum < 373.15
%     y_sat   = CALC_xsat(T_drum);
%     p_vap   = y_sat*p_amb;
%     rho_steam = interp1(T_sat,rho_vap,T_drum,'linear','extrap');
%     p_steam = interp1(T_sat,p_sat,T_drum,'linear','extrap');
%     Z_steam = p_steam.*Mw_water./(rho_steam.*R.*T_drum);
%     M_H2O_v = p_vap.*V_gas./(Z_steam.*R.*T_drum).*Mw_water;
%     x_vap2  = M_H2O_v/M_H2O;
%     a       = (x_vap-x_vap2).*1000;
% else
%     rho_steam = interp1(T_sat,rho_vap,T_drum,'linear','extrap');
%     Z_steam = p.*Mw_water./(rho_steam.*R.*T_drum);
%     N_steam = M_H2O.*x_vap./Mw_water;
%     p_vap   = Z_steam.*N_steam.*R.*T_drum./(V_EVA-(1-x_vap).*M_H2O./rho_water);
%     a       = (p-p_vap);
% end
% Res     = a;
% end
% end

== matlab function Furnace/Plant/Free board/DIFF_Free Board ==
  data: M_fg_int input; dMfg_dt_int output; T_fg input; Fi_in input; T_in input; F_aII input; T_aII input; Q_rad input; p_amb input; dTfg_dt output; Fi_fg_out output; M_fg output; Y_H2O output; V_FreeBoard input; Mw_gas input; T_amb input; cp_fg input; cp_steel input; M_steel_FB input
function [dMfg_dt_int, dTfg_dt,Fi_fg_out,M_fg,Y_H2O] = DIFF_FreeBoard(M_fg_int,T_fg,Fi_in,T_in,F_aII,T_aII,Q_rad,p_amb,V_FreeBoard,Mw_gas,T_amb,cp_fg,cp_steel,M_steel_FB)

% This function calculates the mass and energy balance of the freeboard. The
% furnacefreaboard is treated as one control volume, where the pressure is
% assumed constant in time. 

%%%%%%%%%%%%%%%%%%%%%%%%%%%%%%%%%%%%%%%%%%%%%%%%%%%%%%%%%%%%%%%%%%%%%%%%%%
% Symbol        Units       Explanation
% INPUTS:
% M_fg_int      [kg]        Mass of gas components in the free-board (last
%                           component is missing)
% T_fg          [K]         Temperature flue gas in the free-board
% Fi_in         [kg/s]      Flue gas component mass flows from the grate
% T_in          [K]         Temperature of the flue gas from the grate
% F_aII         [kg/s]      Secondary air mass flow
% T_aII         [K]         Temperature of secondary air 
% Q_rad         [W]         Radiation heat exchanged with the grate
% k              -          Vector of constant parameters
%%%%%%%%%%%%%%%%%%%%%%%%%%%%%%%%%%%%%%%%%%%%%%%%%%%%%%%%%%%%%%%%%%%%%%%%%%

%% Parameters
R           = 8.314462175*1E3;
nc_gas      = size(Fi_in,1);

%%  FLUE GAS  
% Total amount of flue gas in the freeboard is such to have constant p (p=amb)
N_tot       = p_amb.*V_FreeBoard./(R.*T_fg);        % N_tot is used to calculate the amount of the last gas component
N_i         = [M_fg_int./Mw_gas(1:end-1);(N_tot-sum(M_fg_int./Mw_gas(1:end-1)))];  
y_fg        = N_i./N_tot;
Mw_fg       = sum(Mw_gas.*y_fg);
M_fg_tot    = Mw_fg.*N_tot;
M_fg        = N_i.*Mw_gas;
w_fg        = M_fg./M_fg_tot;
Y_H2O       = y_fg(1);

%% INPUTS (functions of time) 
% Gas from grate 
F_in        = sum(Fi_in,1);                         % [kg/s]
w_in        = zeros(size(Fi_in));                   % [kg/kg]
y_in        = zeros(size(Fi_in));
Mw_in       = zeros(size(F_in));
for i = 1:length(F_in)
    w_in(:,i)  = Fi_in(:,i)./F_in(i); 
    y_in(:,i)  = CALC_y_a(w_in(:,i),Mw_gas);        % [kmol/kmol]
    Mw_in(1,i) = sum(Mw_gas.*y_in(:,i));            % [kg/kmol]
end
Q_conv      = sum(F_in.*cp_fg.*(T_in'-T_fg));       % [W]
% Secondary air
w_aII       = CALC_w_ha(T_amb,90,Mw_gas);           % [kg/kg]
Fi_aII      = w_aII.*F_aII;                         % [kg/s]
y_aII       = CALC_y_a(w_aII,Mw_gas);               % [kmol/kmol]
Mw_aII      = sum(Mw_gas.*y_aII);                   % [K]

%% Reaction rates
R_gas       = CALC_Rw_Gas(M_fg,T_fg,nc_gas,Mw_gas,V_FreeBoard);               % [kg/s]
N_gas       = R_gas.R./Mw_gas;                      % [kmol/s]

%% Differential equations
% Temperature equation
dTfg_dt     = 1./(cp_fg.*M_fg_tot+cp_steel.*M_steel_FB).*(Q_conv+F_aII.*cp_fg.*(T_aII-T_fg)+...  	
              R_gas.H+...                                                        
              Q_rad);     
% Time derivative of gas moles in freeboard
dNfg_dt_tot = -N_tot./T_fg.*dTfg_dt;
% Total mole balance
N_out       = sum(F_in./Mw_in) + F_aII./Mw_aII + sum(N_gas) - dNfg_dt_tot;
F_fg_out    = N_out.*Mw_fg;
Fi_fg_out   = F_fg_out.*w_fg;
% Flue gas composition equation
dMfg_dt     = sum(Fi_in,2) + Fi_aII + R_gas.R - Fi_fg_out ;
dMfg_dt_int = dMfg_dt(1:end-1);

== matlab function Furnace/Plant/Gas cleaning systems/SIGURD - Slangefilter ==
  data: T_in input; T_out output; Fi_in input; Fi_solid input; F_kull input; Mw_gas input; Fi_out output; F_ashes output
function [T_out, Fi_out, F_ashes] = fcn(T_in,Fi_in,Fi_solid, F_kull,Mw_gas)


T_out   = T_in;
Fi_out  = Fi_in;
F_ashes = 0;

== matlab function Furnace/Plant/Gas cleaning systems/HeatEx 1 ==
  data: T_in input; T_out output; Fi_in input; T_damp input; epsilon input; Fi_out output; cp_fg input; Q output
function [T_out, Fi_out, Q] = fcn(T_in,Fi_in,  T_damp, epsilon,cp_fg)

% This block is already ready 

F_fg    = sum(Fi_in);
C_min   = cp_fg.*F_fg;
Q       = epsilon.*C_min.*(T_damp-T_in);
T_out   = T_in + Q./(cp_fg.*F_fg);
Fi_out  = Fi_in;

== matlab function Furnace/Plant/Gas cleaning systems/HeatEx 2 ==
  data: T_in input; T_out output; Fi_fg input; Fi_fg output; T2_in input; Fi_fg2 input; epsilon input; eff input; T2_out output; Fi_fg2 output; cp_fg input; Q_loss output
function [T_out, Fi_fg,T2_out, Fi_fg2,Q_loss] = fcn(T_in,Fi_fg, T2_in,Fi_fg2, epsilon,eff,cp_fg)

% This block is already ready 

F_fg1   = sum(Fi_fg);
F_fg2   = sum(Fi_fg2);
C_min   = cp_fg.*min(F_fg1,F_fg2);
Q       = epsilon.*C_min.*(T2_in-T_in);
T_out   = T_in + Q./(cp_fg.*F_fg1);
T2_out  = T2_in- Q./eff./(cp_fg.*F_fg2);
Q_loss  = (1-eff).*Q./eff;

== matlab function Furnace/Plant/Gas cleaning systems/HeatEx 3 ==
  data: T_in input; T_out output; Fi_fg input; T_damp input; Fi_fg output; Q output; epsilon input; cp_fg input
function [T_out, Fi_fg, Q] = fcn(T_in,Fi_fg,  T_damp,epsilon,cp_fg)

% This block is already ready 

F_fg    = sum(Fi_fg);
C_min   = cp_fg.*F_fg;
Q       = epsilon.*C_min.*(T_damp-T_in);
T_out   = T_in + Q./(cp_fg.*F_fg);

== matlab function Furnace/Plant/Gas cleaning systems/SIGURD - SCR (Katalisator) ==
  data: T_in input; T_out output; Fi_fg input; Fi_fg output; F_NH3 input; Mw_gas input
function [T_out, Fi_fg] = fcn(T_in,Fi_fg, F_NH3,Mw_gas)

%%%%%%%%%%%%%%%%%%%%%%%%%%%%%%%%%%%%%%%%%%%%%%%%%%%%%%%%%%%%%%%%%%%%%%%%%%
% INPUTS:
% T_in      [K]         Temperature of the inlet flue gas
% Fi_in     [kg/s]      Vector of mass flow of the gas components
% F_kalk    [kg/s]      Mass flow of kalk
% Mw_gas    [kg/kmol]   Vector of molar masses of the gas components

T_out   = T_in;

== matlab function Furnace/Plant/Turbine/Turbine ==
  data: T_SH input; F_SH input; p_drum input; W_el output; p_HP input; p_LP input; Q_turb output; eta_TURB input
function [W_el, Q_turb ]  = CALC_Turbine(T_SH,F_SH,p_drum,p_HP,p_LP,eta_TURB)

% This function calculates the heat exchanged in the economizer
[p_sat,T_sat,~,~,h_vap,c_p] = SatWater;
cp_vap  = interp1(p_sat,c_p,p_drum,'linear','extrap');
h_sat   = interp1(p_sat,h_vap,p_drum,'linear','extrap');
T_drum  = interp1(p_sat,T_sat,p_drum,'linear','extrap');
h_in    = h_sat + cp_vap.*(T_SH - T_drum);
h_HP    = interp1(p_sat,h_vap,p_HP,'linear','extrap');
% h_LP    = interp1(p_sat,h_vap,p_LP,'linear','extrap');
Q_in    = F_SH.*(h_in - h_HP);
W_el    = eta_TURB.*Q_in;
Q_turb  = (1-eta_TURB).*Q_in;

% % This function calculates the heat exchanged in the economizer
% [p_sat,T_sat,~,~,h_vap,c_p] = SatWater;
% cp_vap  = interp1(p_sat,c_p,p_drum,'linear','extrap');
% h_sat   = interp1(p_sat,h_vap,p_drum,'linear','extrap');
% T_drum  = interp1(p_sat,T_sat,p_drum,'linear','extrap');
% h_in    = h_sat + cp_vap.*(T_SH - T_drum);
% Q_in    = F_SH.*(cp_vap.*(T_SH-T_cond) - H_eva);
% eta_TURB= 32.74 - 0.026.*(T_toDH - 273.15) - 0.089.*(T_fromDH - 273.15);
% W_el    = eta_TURB.*Q_in./100;
% T_turb  = T_cond;

== matlab function Furnace/Plant/Gas cleaning systems/HeatEx 4 ==
  data: T_in input; T_out output; Fi_fg input; Fi_fg output; T2_in input; Fi_fg2 input; epsilon input; T2_out output; Fi_fg2 output; cp_fg input
function [T_out, Fi_fg,T2_out, Fi_fg2] = fcn(T_in,Fi_fg, T2_in,Fi_fg2, epsilon,cp_fg)


F_fg1   = sum(Fi_fg);
F_fg2   = sum(Fi_fg2);
C_min   = cp_fg.*min(F_fg1,F_fg2);
Q       = epsilon.*C_min.*(T_in-T2_in);
T_out   = T_in - Q./(cp_fg.*F_fg1);
T2_out  = T2_in+ Q./(cp_fg.*F_fg2);

== matlab function Furnace/Plant/Gas cleaning systems/SIGURD - Scrubber ==
  data: T_in input; T_out output; Fi_in input; Fi_out output; F_NH3 input; Mw_gas input
function [T_out, Fi_out] = fcn(T_in,Fi_in, F_NH3,Mw_gas)

%%%%%%%%%%%%%%%%%%%%%%%%%%%%%%%%%%%%%%%%%%%%%%%%%%%%%%%%%%%%%%%%%%%%%%%%%%
% INPUTS:
% T_in      [K]         Temperature of the inlet flue gas
% Fi_in     [kg/s]      Vector of mass flow of the gas components
% F_kalk    [kg/s]      Mass flow of kalk
% Mw_gas    [kg/kmol]   Vector of molar masses of the gas components


T_out   = T_in;
Fi_out  = Fi_in;

== matlab function Furnace/Plant/Flue-gas fan/Fan ==
  data: T_fg input; T_out output; F_fg input; W_el output
function [T_out, W_el] = fcn(T_fg,F_fg)

T_out = T_fg;
W_el = 0;

== matlab function Furnace/Waste and Primary air/Input selector ==
  data: constant input; signal output; experimental input; controlled input; input_type input
function signal = ChooseSignal(constant, experimental, controlled, input_type)
    switch(input_type)
        case InputType.Experimental
            signal = experimental;
        case InputType.Controlled
            signal = controlled;
        otherwise
            signal = constant;
    end
end

== matlab function Furnace/Secondary air/Input  selector ==
  data: constant input; signal output; experimental input; controlled input; input_type input
function signal = ChooseSignal(constant, experimental, controlled, input_type)
    switch(input_type)
        case InputType.Experimental
            signal = experimental;
        case InputType.Controlled
            signal = controlled;
        otherwise
            signal = constant;
    end
end

== matlab function Furnace/Plant/Boiler/MATLAB Function ==
  data: p_drum input; k_p_drum input; switch_on output
function switch_on = calc_swch(p_drum, k_p_drum)

switch_on = 0;
if p_drum >= k_p_drum
    switch_on = 1;
end

== matlab function Furnace/Secondary air/Input  selector1 ==
  data: constant input; signal output; experimental input; controlled input; input_type input
function signal = ChooseSignal(constant, experimental, controlled, input_type)
    switch(input_type)
        case InputType.Experimental
            signal = experimental;
        case InputType.Controlled
            signal = controlled;
        otherwise
            signal = constant;
    end
end

== matlab function Furnace/Waste and Primary air/Input selector1 ==
  data: constant input; signal output; experimental input; controlled input; input_type input
function signal = ChooseSignal(constant, experimental, controlled, input_type)
    switch(input_type)
        case InputType.Experimental
            signal = experimental;
        case InputType.Controlled
            signal = controlled;
        otherwise
            signal = constant;
    end
end

== matlab function Furnace/Waste and Primary air/Input selector2 ==
  data: constant input; signal output; experimental input; controlled input; input_type input
function signal = ChooseSignal(constant, experimental, controlled, input_type)
    switch(input_type)
        case InputType.Experimental
            signal = experimental;
        case InputType.Controlled
            signal = controlled;
        otherwise
            signal = constant;
    end
end

== matlab function Furnace/Grate speed/Input selector1 ==
  data: constant input; signal output; experimental input; controlled input; input_type input
function signal = ChooseSignal(constant, experimental, controlled, input_type)
    switch(input_type)
        case InputType.Experimental
            signal = experimental;
        case InputType.Controlled
            signal = controlled;
        otherwise
            signal = constant;
    end
end

== matlab function Furnace/Waste and Primary air/Input selector3 ==
  data: constant input; signal output; experimental input; controlled input; input_type input
function signal = ChooseSignal(constant, experimental, controlled, input_type)
    switch(input_type)
        case InputType.Experimental
            signal = experimental;
        case InputType.Controlled
            signal = controlled;
        otherwise
            signal = constant;
    end
end

== matlab function Furnace/Controller/Input  selector1 ==
  data: constant input; signal output; experimental input; controlled input; input_type input
function signal = ChooseSignal(constant, experimental, controlled, input_type)
    switch(input_type)
        case InputType.Experimental
            signal = experimental;
        case InputType.Controlled
            signal = controlled;
        otherwise
            signal = constant;
    end
end

== matlab function Furnace/Plant/Gas cleaning systems/SIGURD - Reaktor ==
  data: T_in input; T_out output; Fi_in input; F_flyash input; Fi_out output; F_kalk input; Mw_gas input; cp_fg input; F_solid output; F_H2O input
function [T_out, Fi_out, F_solid] = fcn(T_in,Fi_in, F_flyash,F_kalk,Mw_gas,cp_fg, F_H2O)

%%%%%%%%%%%%%%%%%%%%%%%%%%%%%%%%%%%%%%%%%%%%%%%%%%%%%%%%%%%%%%%%%%%%%%%%%%
% INPUTS:
% T_in      [K]         Temperature of the inlet flue gas
% Fi_in     [kg/s]      Vector of mass flow of the gas components
% F_kalk    [kg/s]      Mass flow of kalk
% Mw_gas    [kg/kmol]   Vector of molar masses of the gas components


T_out   = T_in;
Fi_out  = Fi_in;
% The total amount of solid particles equals the flow of flyashes that 
% follow the gas from the combustion chamber + the solid phase particles 
% that form in the reactor
F_solid = F_flyash + 0;

== matlab function Furnace/Controller/Input  selector ==
  data: constant input; signal output; experimental input; controlled input; input_type input
function signal = ChooseSignal(constant, experimental, controlled, input_type)
    switch(input_type)
        case InputType.Experimental
            signal = experimental;
        case InputType.Controlled
            signal = controlled;
        otherwise
            signal = constant;
    end
end

== matlab function Furnace/Controller/Controller selector  ==
  data: ab input; cascade input; signal output; mpc input; controller_type input
function signal = ChooseController(ab, cascade, mpc, controller_type)
   
switch(controller_type)
        case ControllerType.AB
            signal = ab;
        case ControllerType.Cascade
            signal = cascade;
        otherwise
            signal = mpc;
    end
end

== matlab function Furnace/Controller/Controller selector 1 ==
  data: ab input; cascade input; signal output; mpc input; controller_type input
function signal = ChooseController(ab, cascade, mpc, controller_type)
   
switch(controller_type)
        case ControllerType.AB
            signal = ab;
        case ControllerType.Cascade
            signal = cascade;
        otherwise
            signal = mpc;
    end
end

== matlab function Furnace/Controller/Controller selector 2 ==
  data: ab input; cascade input; signal output; mpc input; controller_type input
function signal = ChooseController(ab, cascade, mpc, controller_type)
   
switch(controller_type)
        case ControllerType.AB
            signal = ab;
        case ControllerType.Cascade
            signal = cascade;
        otherwise
            signal = mpc;
    end
end

== matlab function Furnace/Controller/Controller selector 3 ==
  data: ab input; cascade input; signal output; mpc input; controller_type input
function signal = ChooseController(ab, cascade, mpc, controller_type)
   
switch(controller_type)
        case ControllerType.AB
            signal = ab;
        case ControllerType.Cascade
            signal = cascade;
        otherwise
            signal = mpc;
    end
end
